simulink model "suspension_shaker_rig"  (R2024b)
settings: Solver=FixedStepAuto  StartTime=0.0  StopTime=100  FixedStep=0.001  RelTol=1e-3
values from neighbouring files (symbols this model uses):
  A = 1.25    [final_par.m]
  a = 1.80    (= 1.8)    [final_par.m]
  b = L-a    (= 1.7)    [final_par.m]
  cdf = 1400.00    (= 1400)    [final_par.m]
  cdr = 1800.00    (= 1800)    [final_par.m]
  cz = 1.00    (= 1)    [final_par.m]
  F0fl = ms*g*(b/L)*1/2    (= 1870.20642857)    [final_par.m]
  F0fr = F0fl    (= 1870.20642857)    [final_par.m]
  F0rl = ms*g*(a/L)*1/2    (= 1980.21857143)    [final_par.m]
  F0rr = F0rl    (= 1980.21857143)    [final_par.m]
  g = 9.81    [final_par.m]
  hrcf = 0.04    [final_par.m]
  hrcr = 0.06    [final_par.m]
  Ixx = 300.00    (= 300)    [final_par.m]
  Iyy = 1350.00    (= 1350)    [final_par.m]
  kARBf = 5000.00    (= 5000)    [final_par.m]
  kARBr = 1000.00    (= 1000)    [final_par.m]
  ksf = 67500.00    (= 67500)    [final_par.m]
  ksr = 100000.00    (= 100000)    [final_par.m]
  ktyre = 400000.00    (= 400000)    [final_par.m]
  L = 3.50    (= 3.5)    [final_par.m]
  ms = m-2*musf-2*musr    (= 785)    [final_par.m]
  musf = 15.00    (= 15)    [final_par.m]
  musr = 17.50    (= 17.5)    [final_par.m]
  r = 0.375    [final_par.m]
  rho = 1.225    [final_par.m]
  tr = 1.85    [final_par.m]
  z0tfl = (ms*(b/L)*1/2+musf)*g/ktyre    (= 0.00504339107143)    [final_par.m]
  z0tfr = z0tfl    (= 0.00504339107143)    [final_par.m]
  z0trl = (ms*(a/L)*1/2+musr)*g/ktyre    (= 0.00537973392857)    [final_par.m]
  z0trr = z0trl    (= 0.00537973392857)    [final_par.m]
libraries: simulink x1
settings Model: Creator=ravas  LastModifiedBy=ravas
settings DataIOCC: ReturnWorkspaceOutputs=off

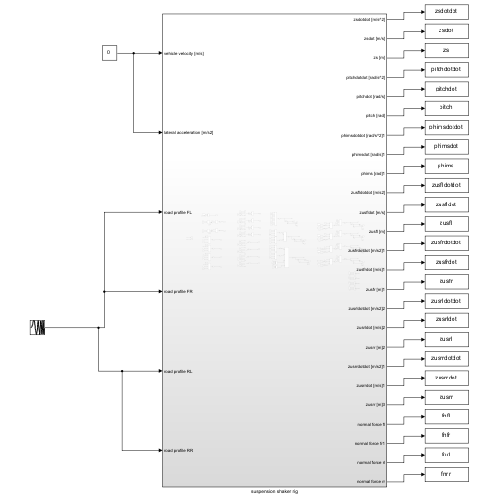
[thumbnail: Simulink's stored preview of the top-level diagram]
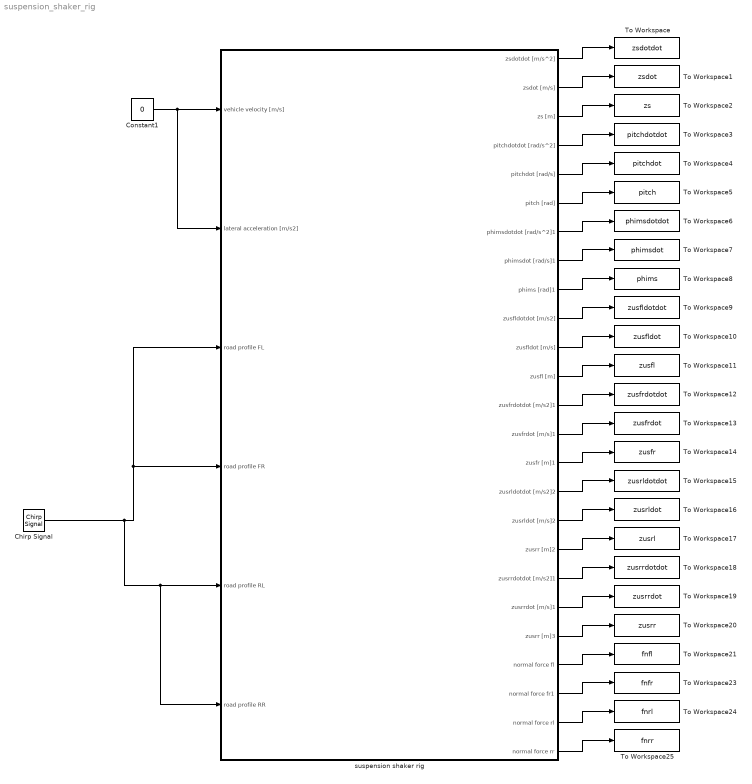
== system suspension_shaker_rig ==
  Chirp Signal : simulink/Sources/Chirp Signal  f1=0.1  T=100  f2=50
  Constant1 : Constant  Value=0
  To Workspace : ToWorkspace  VariableName=zsdotdot  SaveFormat=Timeseries  SampleTime=-1
  To Workspace1 : ToWorkspace  VariableName=zsdot  SaveFormat=Timeseries  SampleTime=-1
  To Workspace10 : ToWorkspace  VariableName=zusfldot  SaveFormat=Timeseries  SampleTime=-1
  To Workspace11 : ToWorkspace  VariableName=zusfl  SaveFormat=Timeseries  SampleTime=-1
  To Workspace12 : ToWorkspace  VariableName=zusfrdotdot  SaveFormat=Timeseries  SampleTime=-1
  To Workspace13 : ToWorkspace  VariableName=zusfrdot  SaveFormat=Timeseries  SampleTime=-1
  To Workspace14 : ToWorkspace  VariableName=zusfr  SaveFormat=Timeseries  SampleTime=-1
  To Workspace15 : ToWorkspace  VariableName=zusrldotdot  SaveFormat=Timeseries  SampleTime=-1
  To Workspace16 : ToWorkspace  VariableName=zusrldot  SaveFormat=Timeseries  SampleTime=-1
  To Workspace17 : ToWorkspace  VariableName=zusrl  SaveFormat=Timeseries  SampleTime=-1
  To Workspace18 : ToWorkspace  VariableName=zusrrdotdot  SaveFormat=Timeseries  SampleTime=-1
  To Workspace19 : ToWorkspace  VariableName=zusrrdot  SaveFormat=Timeseries  SampleTime=-1
  To Workspace2 : ToWorkspace  VariableName=zs  SaveFormat=Timeseries  SampleTime=-1
  To Workspace20 : ToWorkspace  VariableName=zusrr  SaveFormat=Timeseries  SampleTime=-1
  To Workspace21 : ToWorkspace  VariableName=fnfl  SaveFormat=Timeseries  SampleTime=-1
  To Workspace23 : ToWorkspace  VariableName=fnfr  SaveFormat=Timeseries  SampleTime=-1
  To Workspace24 : ToWorkspace  VariableName=fnrl  SaveFormat=Timeseries  SampleTime=-1
  To Workspace25 : ToWorkspace  VariableName=fnrr  SaveFormat=Timeseries  SampleTime=-1
  To Workspace3 : ToWorkspace  VariableName=pitchdotdot  SaveFormat=Timeseries  SampleTime=-1
  To Workspace4 : ToWorkspace  VariableName=pitchdot  SaveFormat=Timeseries  SampleTime=-1
  To Workspace5 : ToWorkspace  VariableName=pitch  SaveFormat=Timeseries  SampleTime=-1
  To Workspace6 : ToWorkspace  VariableName=phimsdotdot  SaveFormat=Timeseries  SampleTime=-1
  To Workspace7 : ToWorkspace  VariableName=phimsdot  SaveFormat=Timeseries  SampleTime=-1
  To Workspace8 : ToWorkspace  VariableName=phims  SaveFormat=Timeseries  SampleTime=-1
  To Workspace9 : ToWorkspace  VariableName=zusfldotdot  SaveFormat=Timeseries  SampleTime=-1
  suspension shaker rig : Subsystem
  wires:
  suspension shaker rig/1(zsdotdot [m/s^2]) -> To Workspace/1
  suspension shaker rig/2(zsdot [m/s]) -> To Workspace1/1
  suspension shaker rig/3(zs [m]) -> To Workspace2/1
  suspension shaker rig/4(pitchdotdot [rad/s^2]) -> To Workspace3/1
  suspension shaker rig/5(pitchdot [rad/s]) -> To Workspace4/1
  suspension shaker rig/6(pitch [rad]) -> To Workspace5/1
  suspension shaker rig/7(phimsdotdot [rad/s^2]1) -> To Workspace6/1
  suspension shaker rig/8(phimsdot [rad/s]1) -> To Workspace7/1
  suspension shaker rig/9(phims [rad]1) -> To Workspace8/1
  suspension shaker rig/10(zusfldotdot [m/s2]) -> To Workspace9/1
  suspension shaker rig/11(zusfldot [m/s]) -> To Workspace10/1
  suspension shaker rig/12(zusfl [m]) -> To Workspace11/1
  suspension shaker rig/13(zusfrdotdot [m/s2]1) -> To Workspace12/1
  suspension shaker rig/14(zusfrdot [m/s]1) -> To Workspace13/1
  suspension shaker rig/15(zusfr [m]1) -> To Workspace14/1
  suspension shaker rig/16(zusrldotdot [m/s2]2) -> To Workspace15/1
  suspension shaker rig/17(zusrldot [m/s]2) -> To Workspace16/1
  suspension shaker rig/18(zusrr [m]2) -> To Workspace17/1
  suspension shaker rig/19(zusrrdotdot [m/s2]1) -> To Workspace18/1
  suspension shaker rig/20(zusrrdot [m/s]1) -> To Workspace19/1
  suspension shaker rig/21(zusrr [m]3) -> To Workspace20/1
  suspension shaker rig/22(normal force fl) -> To Workspace21/1
  suspension shaker rig/23(normal force fr1) -> To Workspace23/1
  suspension shaker rig/24(normal force rl) -> To Workspace24/1
  suspension shaker rig/25(normal force rr) -> To Workspace25/1
  Constant1/1 -> suspension shaker rig/2(lateral acceleration [m/s2]), suspension shaker rig/1(vehicle velocity [m/s])
  Chirp Signal/1 -> suspension shaker rig/6(road profile RR), suspension shaker rig/5(road profile RL), suspension shaker rig/4(road profile FR), suspension shaker rig/3(road profile FL)

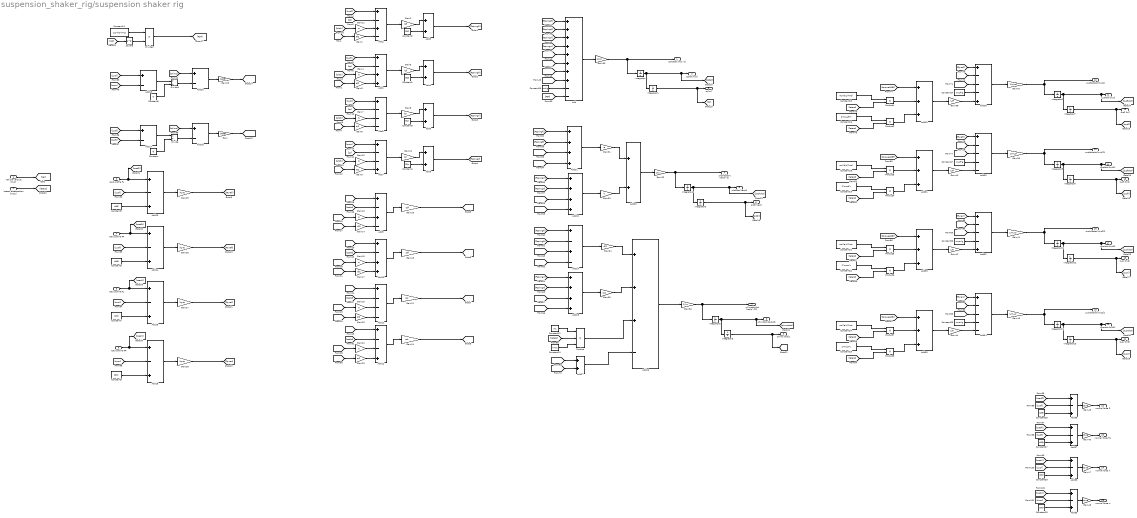
== system suspension_shaker_rig/suspension shaker rig ==
  vehicle velocity [m/s] : Inport
  lateral acceleration [m/s2] : Inport  Port=2
  road profile FL : Inport  Port=3
  road profile FR : Inport  Port=4
  road profile RL : Inport  Port=5
  road profile RR : Inport  Port=6
  Add : Sum  Inputs=++++++++--
  Add1 : Sum  Inputs=+-++
  Add10 : Sum  Inputs=+-++
  Add11 : Sum  Inputs=+---
  Add12 : Sum  Inputs=+--+
  Add{13..16,36..39} (8 alike) : Sum  Inputs=+-+
  Add{17..20} (4 alike) : Sum  Inputs=+-
  Add2 : Sum  Inputs=+-+-
  Add21 : Sum  Inputs=++++
  Add22 : Sum  Inputs=++++
  Add{3..4,6,8,23,27} (6 alike) : Sum
  Add24 : Sum  Inputs=+-+-
  Add25 : Sum  Inputs=++++
  Add26 : Sum  Inputs=+++-
  Add28 : Sum  Inputs=+---+
  Add{29,31,33,35} (4 alike) : Sum  Inputs=+++
  Add30 : Sum  Inputs=+----
  Add32 : Sum  Inputs=+---+
  Add34 : Sum  Inputs=+----
  Add5 : Sum  Inputs=+---
  Add7 : Sum  Inputs=+--+
  Add9 : Sum  Inputs=+-+-
  Constant : Constant  Value=tf
  Constant1 : Constant  Value=F0fr
  Constant10 : Constant  Value=ms*g
  Constant11 : Constant  Value=1/2*rho*A*cz
  Constant12 : Constant  Value=ms
  Constant13 : Constant  Value=h-hrc
  Constant14 : Constant  Value=musf*g
  Constant15 : Constant  Value=ms*(b/L)*hrcf
  Constant16 : Constant  Value=2*(musf)*r
  Constant17 : Constant  Value=musf*g
  Constant18 : Constant  Value=ms*(b/L)*hrcf
  Constant19 : Constant  Value=2*musf*r
  Constant2 : Constant  Value=F0fl
  Constant20 : Constant  Value=musr*g
  Constant21 : Constant  Value=ms*(a/L)*hrcr
  Constant22 : Constant  Value=2*musr*r
  Constant23 : Constant  Value=musr*g
  Constant24 : Constant  Value=ms*(a/L)*hrcr
  Constant25 : Constant  Value=2*musr*r
  Constant26 : Constant  Value=z0tfl
  Constant27 : Constant  Value=z0tfr
  Constant28 : Constant  Value=z0trl
  Constant29 : Constant  Value=z0trr
  Constant3 : Constant  Value=F0rl
  Constant4 : Constant  Value=F0rr
  Constant5 : Constant  Value=z0tfl
  Constant6 : Constant  Value=z0tfr  VectorParams1D=off
  Constant7 : Constant  Value=z0trl  VectorParams1D=off
  Constant8 : Constant  Value=z0trr  VectorParams1D=off
  Constant9 : Constant  Value=tr
  Divide : Product  Inputs=*/
  Divide1 : Product  Inputs=*/
  Divide2 : Product  Inputs=**
  Gain : Gain  Gain=kARBf
  Gain{1,3,14,17,34} (5 alike) : Gain  Gain=tf/2
  Gain{7,10,19,22,33} (5 alike) : Gain  Gain=b
  Gain{4,11,13,15} (4 alike) : Gain  Gain=a
  Gain12 : Gain  Gain=ksr
  Gain16 : Gain  Gain=cdf
  Gain18 : Gain  Gain=cdf
  Gain2 : Gain  Gain=ksf
  Gain{6,9,20,23,35} (5 alike) : Gain  Gain=tr/2
  Gain21 : Gain  Gain=cdr
  Gain24 : Gain  Gain=cdr
  Gain{25..28,45..48} (8 alike) : Gain  Gain=ktyre
  Gain29 : Gain  Gain=kARBr
  Gain30 : Gain  Gain=1/ms
  Gain31 : Gain  Gain=-a
  Gain32 : Gain  Gain=1/Iyy
  Gain36 : Gain  Gain=1/Ixx
  Gain37 : Gain  Gain=1/musf
  Gain38 : Gain  Gain=1/tf
  Gain39 : Gain  Gain=1/musf
  Gain40 : Gain  Gain=1/tf
  Gain41 : Gain  Gain=1/musr
  Gain42 : Gain  Gain=1/tr
  Gain43 : Gain  Gain=1/musr
  Gain44 : Gain  Gain=1/tr
  Gain5 : Gain  Gain=ksf
  Gain8 : Gain  Gain=ksr
  Integrator{,1..13} (14 alike) : Integrator
  Product : Product  Inputs=3
  Product{1..8} (8 alike) : Product
  Square : Math  Operator=square
  zsdotdot [m/s^2] : Outport
  zsdot [m/s] : Outport  Port=2
  zs [m] : Outport  Port=3
  pitchdotdot [rad/s^2] : Outport  Port=4
  pitchdot [rad/s] : Outport  Port=5
  pitch [rad] : Outport  Port=6
  phimsdotdot [rad/s^2]1 : Outport  Port=7
  phimsdot [rad/s]1 : Outport  Port=8
  phims [rad]1 : Outport  Port=9
  zusfldotdot [m/s2] : Outport  Port=10
  zusfldot [m/s] : Outport  Port=11
  zusfl [m] : Outport  Port=12
  zusfrdotdot [m/s2]1 : Outport  Port=13
  zusfrdot [m/s]1 : Outport  Port=14
  zusfr [m]1 : Outport  Port=15
  zusrldotdot [m/s2]2 : Outport  Port=16
  zusrldot [m/s]2 : Outport  Port=17
  zusrr [m]2 : Outport  Port=18
  zusrrdotdot [m/s2]1 : Outport  Port=19
  zusrrdot [m/s]1 : Outport  Port=20
  zusrr [m]3 : Outport  Port=21
  normal force fl : Outport  Port=22
  normal force fr1 : Outport  Port=23
  normal force rl : Outport  Port=24
  normal force rr : Outport  Port=25
  wires:
  [zusfl] -> Add2/1
  Add2/1 -> Gain2/1
  Gain11/1 -> Add2/3
  [zs] -> Add2/2
  Constant2/1 -> Add3/2
  [pitch] -> Gain11/1
  Gain2/1 -> Add3/1
  Add3/1 -> [Fspringfl]  "front left spring force [N]"
  [phims] -> Gain1/1
  Gain1/1 -> Add2/4
  Gain5/1 -> Add4/1
  [pitch] -> Gain4/1
  [zusfr] -> Add1/1
  Add4/1 -> [Fspringfr]  "front right spring force [N]"
  [zs] -> Add1/2
  Constant1/1 -> Add4/2
  Add1/1 -> Gain5/1
  Gain4/1 -> Add1/3
  Gain3/1 -> Add1/4
  [phims] -> Gain3/1
  [phims] -> Gain6/1
  Gain6/1 -> Add5/4
  Gain7/1 -> Add5/3
  Add5/1 -> Gain8/1
  Constant3/1 -> Add6/2
  [zs] -> Add5/2
  Add6/1 -> [Fspringrl]  "rear left spring force [N]"
  [zusrl] -> Add5/1
  [pitch] -> Gain7/1
  Gain8/1 -> Add6/1
  Gain12/1 -> Add8/1
  [pitch] -> Gain10/1
  [zusrr] -> Add7/1
  Add8/1 -> [Fspringrr]  "rear right spring force [N]"
  [zs] -> Add7/2
  Constant4/1 -> Add8/2
  Add7/1 -> Gain12/1
  Gain10/1 -> Add7/3
  Gain9/1 -> Add7/4
  [phims] -> Gain9/1
  [zsdot] -> Add9/2
  Gain13/1 -> Add9/3
  [pitchdot] -> Gain13/1
  Gain16/1 -> [Fdamperfl]  "front left damper force"
  Add9/1 -> Gain16/1
  [zusfldot] -> Add9/1
  [phimsdot] -> Gain14/1
  Gain14/1 -> Add9/4
  Gain17/1 -> Add10/4
  [phimsdot] -> Gain17/1
  [zusfrdot] -> Add10/1
  Add10/1 -> Gain18/1
  Gain18/1 -> [Fdamperfr]  "front right damper force"
  [pitchdot] -> Gain15/1
  Gain15/1 -> Add10/3
  [zsdot] -> Add10/2
  [zsdot] -> Add11/2
  Gain19/1 -> Add11/3
  [pitchdot] -> Gain19/1
  Gain21/1 -> [Fdamperrl]  "rear left damper force"
  Add11/1 -> Gain21/1
  [zusrldot] -> Add11/1
  [phimsdot] -> Gain20/1
  Gain20/1 -> Add11/4
  Gain23/1 -> Add12/4
  [phimsdot] -> Gain23/1
  [zusrrdot] -> Add12/1
  Add12/1 -> Gain24/1
  Gain24/1 -> [Fdamperrr]  "rear right damper force"
  [pitchdot] -> Gain22/1
  Gain22/1 -> Add12/3
  [zsdot] -> Add12/2
  Constant5/1 -> Add13/3
  [zusfl] -> Add13/2
  road profile FL/1 -> [roadfl], Add13/1
  Gain25/1 -> [Ftyrefl]  "tyre force [N]"
  Add13/1 -> Gain25/1
  road profile FR/1 -> [roadfr], Add14/1
  Add14/1 -> Gain26/1
  Gain26/1 -> [Ftyrefr]  "tyre force [N]"
  [zusfr] -> Add14/2
  Constant6/1 -> Add14/3
  Constant7/1 -> Add15/3
  Gain27/1 -> [Ftyrerl]  "tyre force [N]"
  road profile RL/1 -> [roadrl], Add15/1
  [zusrl] -> Add15/2
  Add15/1 -> Gain27/1
  Constant8/1 -> Add16/3
  Gain28/1 -> [Ftyrerr]  "tyre force [N]"
  road profile RR/1 -> [roadrr], Add16/1
  [zusrr] -> Add16/2
  Add16/1 -> Gain28/1
  [zusfr] -> Add17/2
  [zusfl] -> Add17/1
  Add17/1 -> Divide/1
  Constant/1 -> Divide/2
  Divide/1 -> Add18/2
  [phims] -> Add18/1
  Add18/1 -> Gain/1
  Gain/1 -> [torqueARBf]
  Add19/1 -> Divide1/1
  Divide1/1 -> Add20/2
  [zusrr] -> Add19/2
  Constant9/1 -> Divide1/2
  Add20/1 -> Gain29/1
  [phims] -> Add20/1
  Gain29/1 -> [torqueARBr]
  [zusrl] -> Add19/1
  [Fspringfr] -> Add/2
  Integrator/1 -> Integrator1/1, [zsdot], zsdot [m/s]/1  "sprung mass vert velocity [m/s]"
  Gain30/1 -> Integrator/1, zsdotdot [m/s^2]/1  "sprung mass vertical acc [m/s2]"
  Integrator1/1 -> [zs], zs [m]/1  "sprung mass vertical displacement"
  [Fspringrr] -> Add/4
  Add/1 -> Gain30/1
  [Fspringrl] -> Add/3
  [Fspringfl] -> Add/1
  [Fdamperfl] -> Add/5
  [Fdamperfr] -> Add/6
  [Fdamperrl] -> Add/7
  [Fdamperrr] -> Add/8
  Constant10/1 -> Add/9
  [FDF] -> Add/10
  Constant11/1 -> Divide2/1
  vehicle velocity [m/s]/1 -> [Vel]
  [Vel] -> Square/1
  Square/1 -> Divide2/2
  Divide2/1 -> [FDF]  "downforce [N]"
  Gain32/1 -> pitchdotdot [rad/s^2]/1, Integrator4/1  "sprung mass pitch acc [rad/s2]"
  Integrator5/1 -> [pitch], pitch [rad]/1  "sprung mass pitch rotation [rad]"
  Integrator4/1 -> Integrator5/1, [pitchdot], pitchdot [rad/s]/1  "sprung mass pitch velocity [rad/s]"
  [Fspringfl] -> Add21/1
  [Fspringfr] -> Add21/2
  [Fdamperfl] -> Add21/3
  [Fdamperfr] -> Add21/4
  Add21/1 -> Gain31/1
  Add22/1 -> Gain33/1
  [Fdamperrr] -> Add22/4
  [Fdamperrl] -> Add22/3
  [Fspringrr] -> Add22/2
  [Fspringrl] -> Add22/1
  Gain31/1 -> Add23/1
  Gain33/1 -> Add23/2
  Add23/1 -> Gain32/1
  [Fdamperfr] -> Add24/4
  [Fdamperfl] -> Add24/3
  [Fspringfr] -> Add24/2
  [Fspringfl] -> Add24/1
  Add24/1 -> Gain34/1
  [Fspringrl] -> Add25/1
  [Fspringrr] -> Add25/2
  [Fdamperrl] -> Add25/3
  [Fdamperrr] -> Add25/4
  Add25/1 -> Gain35/1
  Gain34/1 -> Add26/1
  Gain35/1 -> Add26/2
  lateral acceleration [m/s2]/1 -> [latacc]
  Constant12/1 -> Product/1
  [latacc] -> Product/2
  Constant13/1 -> Product/3
  Product/1 -> Add26/3
  [torqueARBr] -> Add27/2
  [torqueARBf] -> Add27/1
  Add27/1 -> Add26/4
  Gain36/1 -> phimsdotdot [rad/s^2]1/1, Integrator2/1  "sprung mass pitch acc [rad/s2]"
  Integrator3/1 -> [phims], phims [rad]1/1  "sprung mass pitch rotation [rad]"
  Integrator2/1 -> Integrator3/1, [phimsdot], phimsdot [rad/s]1/1  "sprung mass pitch velocity [rad/s]"
  Add26/1 -> Gain36/1
  [Fdamperfl] -> Add28/3
  Gain37/1 -> Integrator6/1, zusfldotdot [m/s2]/1  "front left unsprung mass vertical acc [m/s2]"
  Integrator7/1 -> [zusfl], zusfl [m]/1  "front left unsprung mass vertical displacement [m]"
  [Fspringfl] -> Add28/2
  [Ftyrefl] -> Add28/1
  Add28/1 -> Gain37/1
  Integrator6/1 -> [zusfldot], zusfldot [m/s]/1, Integrator7/1  "front left unsprung mass vert velocity [m/s]"
  Constant14/1 -> Add28/4
  Add29/1 -> Gain38/1
  Gain38/1 -> Add28/5
  [torqueARBf] -> Add29/1
  Constant15/1 -> Product1/1
  [latacc] -> Product1/2
  Product1/1 -> Add29/2
  [latacc] -> Product2/2
  Constant16/1 -> Product2/1
  Product2/1 -> Add29/3
  Product4/1 -> Add31/3
  Constant19/1 -> Product4/1
  [latacc] -> Product4/2
  Product3/1 -> Add31/2
  [latacc] -> Product3/2
  Constant18/1 -> Product3/1
  [torqueARBf] -> Add31/1
  Gain40/1 -> Add30/5
  Add31/1 -> Gain40/1
  Constant17/1 -> Add30/4
  Integrator8/1 -> Integrator9/1, zusfrdot [m/s]1/1, [zusfrdot]  "front right unsprung mass vert velocity [m/s]"
  Add30/1 -> Gain39/1
  [Ftyrefr] -> Add30/1
  [Fspringfr] -> Add30/2
  Integrator9/1 -> zusfr [m]1/1, [zusfr]  "front right unsprung mass vertical displacement [m]"
  Gain39/1 -> zusfrdotdot [m/s2]1/1, Integrator8/1  "front right unsprung mass vertical acc [m/s2]"
  [Fdamperfr] -> Add30/3
  Gain41/1 -> zusrldotdot [m/s2]2/1, Integrator10/1  "rear left unsprung mass vertical acc [m/s2]"
  Integrator11/1 -> zusrr [m]2/1, [zusrl]  "rear left unsprung mass vertical displacement [m]"
  [Fdamperrl] -> Add32/3
  Integrator10/1 -> Integrator11/1, zusrldot [m/s]2/1, [zusrldot]  "rear left unsprung mass vert velocity [m/s]"
  [Ftyrerl] -> Add32/1
  Add32/1 -> Gain41/1
  Constant20/1 -> Add32/4
  [latacc] -> Product6/2
  Gain42/1 -> Add32/5
  Product6/1 -> Add33/3
  [torqueARBr] -> Add33/1
  [latacc] -> Product5/2
  Constant21/1 -> Product5/1
  Constant22/1 -> Product6/1
  Product5/1 -> Add33/2
  [Fspringrl] -> Add32/2
  Add33/1 -> Gain42/1
  Add35/1 -> Gain44/1
  [Fspringrr] -> Add34/2
  Gain44/1 -> Add34/5
  [latacc] -> Product8/2
  [torqueARBr] -> Add35/1
  Add34/1 -> Gain43/1
  Constant23/1 -> Add34/4
  Product8/1 -> Add35/3
  Product7/1 -> Add35/2
  Constant24/1 -> Product7/1
  [Ftyrerr] -> Add34/1
  [latacc] -> Product7/2
  Constant25/1 -> Product8/1
  [Fdamperrr] -> Add34/3
  Integrator12/1 -> Integrator13/1, zusrrdot [m/s]1/1, [zusrrdot]  "rear right unsprung mass vert velocity [m/s]"
  Gain43/1 -> zusrrdotdot [m/s2]1/1, Integrator12/1  "rear right unsprung mass vertical acc [m/s2]"
  Integrator13/1 -> zusrr [m]3/1, [zusrr]  "rear right unsprung mass vertical displacement [m]"
  Add36/1 -> Gain45/1
  Gain45/1 -> normal force fl/1
  [roadfl] -> Add36/1
  [zusfl] -> Add36/2
  Constant26/1 -> Add36/3
  [zusfr] -> Add37/2
  [roadfr] -> Add37/1
  Gain46/1 -> normal force fr1/1
  Constant27/1 -> Add37/3
  Add37/1 -> Gain46/1
  Gain47/1 -> normal force rl/1
  Constant28/1 -> Add38/3
  Add38/1 -> Gain47/1
  [roadrl] -> Add38/1
  [zusrl] -> Add38/2
  [zusrr] -> Add39/2
  Constant29/1 -> Add39/3
  [roadrr] -> Add39/1
  Add39/1 -> Gain48/1
  Gain48/1 -> normal force rr/1
